simulink model "LQI_Controller"  (R2025a)
settings: Solver=FixedStepDiscrete  StartTime=0.0  StopTime=2000  FixedStep=0.01  RelTol=1e-3
values from neighbouring files (symbols this model uses):
  Ke_d = [-0.0924393948471  -0.00817730128246; 0.00819789025598  -0.0924279791075]    [LQI_params.mat]    (also in main_control.m = K_aug_d(:, 5:6))
  Kx_d = [0.12575397263  0.814001770908  0.0258937320835  0.0687846498717; -0.0126880421789  -0.0790152821896  0.235851467161  0.775518858724]    [LQI_params.mat]    (also in main_control.m = K_aug_d(:, 1:4))
  u_bar = [6.60003195923 9.28189672086]    [LQI_params.mat]    (also in linearize_4tanks.m = reshape(z_opt(5:6), [2, 1]))
  x_bar = [24.6597369405 10 3.03378366821 10]    [LQI_params.mat]    (also in linearize_4tanks.m = reshape(z_opt(1:4), [4, 1]))
  xv = 0:0.05:18    [main_control.m]
  ygamma1 = gamma1_fcn(xv)    [main_control.m]
  ygamma2 = gamma2_fcn(xv)    [main_control.m]
  yk1 = k1_fcn(xv)    [main_control.m]
  yk2 = k2_fcn(xv)    [main_control.m]
undefined symbols (not defined in the file or in its folder): AA, DiscIntNeverNeededParam
libraries: simulink x2, simulink_extras x2
settings Model: Creator=oguzhanenes  LastModifiedBy=oguzhanenes

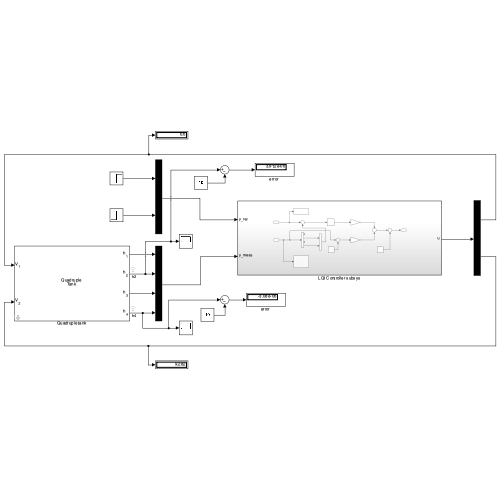
[thumbnail: Simulink's stored preview of the top-level diagram]
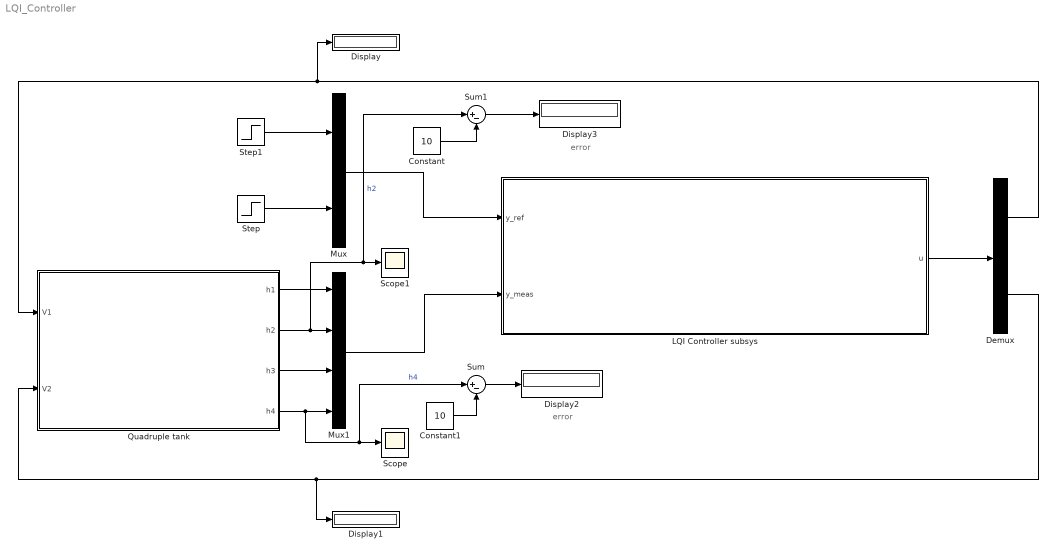
== system LQI_Controller ==
  note: error
  note: error
  Constant : Constant  Value=10
  Constant1 : Constant  Value=10
  Demux : Demux  Outputs=2
  Display{,1..3} (4 alike) : Display
  LQI Controller subsys : Subsystem
  Mux : Mux  Inputs=2
  Mux1 : Mux
  Quadruple tank : Subsystem  mask{h_0=x_bar, A=AA, S=(4.44 / 2)^2 * pi * ones(1, 4), g=981}
      mask prompts: h_0 "Initial level"; A "Outlet section"; S "Tank section"; g "Gravity"
      mask DialogControl h_0 Tooltip: [cm]
      mask DialogControl A Tooltip: [cm^2]
      mask DialogControl S Tooltip: [cm^2]
      mask DialogControl g Tooltip: [cm/s^2]
      mask Display:
      | disp('Quadruple\nTank');
      | port_label('input', 1, 'V_1', 'interpreter', 'tex');
      | port_label('input', 2, 'V_2', 'interpreter', 'tex');
      | port_label('output', 1, 'h_1', 'interpreter', 'tex');
      | port_label('output', 2, 'h_2', 'interpreter', 'tex');
      | port_label('output', 3, 'h_3', 'interpreter', 'tex');
      | port_label('output', 4, 'h_4', 'interpreter', 'tex');
  Scope : Scope
      settings: ActiveDisplayYMinimum=-838.37574082591277  ActiveDisplayYMaximum=411.67749053415992
  Scope1 : Scope
      settings: ActiveDisplayYMinimum=9.94619790425928  ActiveDisplayYMaximum=10.03798510174054
  Step : Step  Time=500  Before=10  After=10  SampleTime=0
  Step1 : Step  Time=500  Before=10  After=10  SampleTime=0
  Sum : Sum  Inputs=|+-
  Sum1 : Sum  Inputs=|+-
  wires:
  Step/1 -> Mux/2
  Mux1/1 -> LQI Controller subsys/2(y_meas)
  Mux/1 -> LQI Controller subsys/1(y_ref)
  Step1/1 -> Mux/1
  LQI Controller subsys/1(u) -> Demux/1
  Quadruple tank/1(h1) -> Mux1/1
  Quadruple tank/2(h2) -> Sum1/1, Scope1/1, Mux1/2  "h2"
  Quadruple tank/3(h3) -> Mux1/3
  Quadruple tank/4(h4) -> Sum/1, Scope/1, Mux1/4  "h4"
  Demux/1 -> Display/1, Quadruple tank/1(V1)
  Demux/2 -> Quadruple tank/2(V2), Display1/1
  Sum1/1 -> Display3/1
  Constant/1 -> Sum1/2
  Constant1/1 -> Sum/2
  Sum/1 -> Display2/1

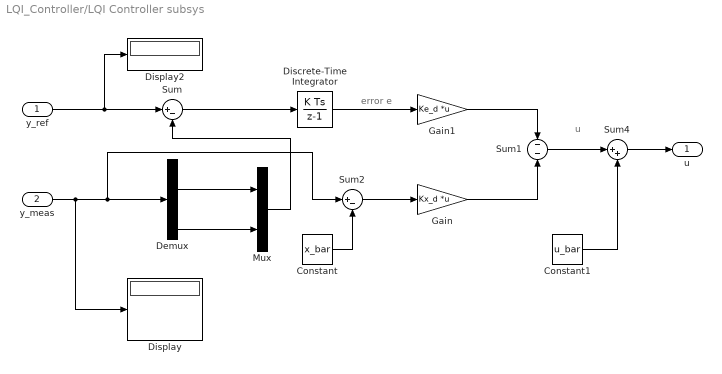
== system LQI_Controller/LQI Controller subsys ==
  note: u
  note: error e
  y_ref : Inport
  y_meas : Inport  Port=2
  Constant : Constant  Value=x_bar
  Constant1 : Constant  Value=u_bar
  Demux : Demux
  Discrete-Time Integrator : DiscreteIntegrator  SampleTime=0.01  ICPrevOutput=DiscIntNeverNeededParam  ICPrevScaledInput=DiscIntNeverNeededParam
  Display : Display
  Display2 : Display
  Gain : Gain  Gain=Kx_d  Multiplication=Matrix(K*u) (u vector)
  Gain1 : Gain  Gain=Ke_d  Multiplication=Matrix(K*u) (u vector)
  Mux : Mux  Inputs=2
  Sum : Sum  Inputs=|+-
  Sum1 : Sum  Inputs=--
  Sum2 : Sum  Inputs=|+-
  Sum4 : Sum  Inputs=|++
  u : Outport
  wires:
  y_ref/1 -> Display2/1, Sum/1
  Discrete-Time Integrator/1 -> Gain1/1
  Gain/1 -> Sum1/2
  Constant1/1 -> Sum4/2
  Sum1/1 -> Sum4/1
  Sum4/1 -> u/1
  y_meas/1 -> Display/1, Sum2/1, Demux/1
  Demux/2 -> Mux/1
  Demux/4 -> Mux/2
  Mux/1 -> Sum/2
  Sum2/1 -> Gain/1
  Constant/1 -> Sum2/2
  Gain1/1 -> Sum1/1
  Sum/1 -> Discrete-Time Integrator/1

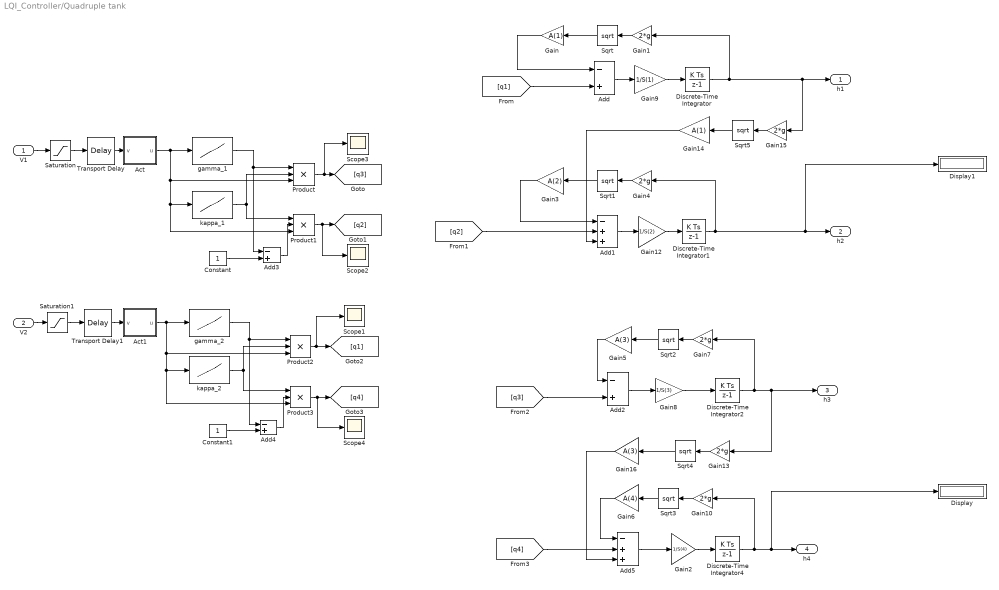
== system LQI_Controller/Quadruple tank ==
  V1 : Inport
  V2 : Inport  Port=2
  Act : Subsystem
  Act1 : Subsystem
  Add{,2..4} (4 alike) : Sum  Inputs=-+
  Add1 : Sum  Inputs=-++
  Add5 : Sum  Inputs=-++
  Constant : Constant
  Constant1 : Constant
  Discrete-Time Integrator{,1..2,4} (4 alike) : DiscreteIntegrator  SampleTime=0.01  ICPrevOutput=DiscIntNeverNeededParam  ICPrevScaledInput=DiscIntNeverNeededParam
  Display : Display
  Display1 : Display
  Gain : Gain  Gain=A(1)
  Gain{1,4,7,10,13,15} (6 alike) : Gain  Gain=2*g
  Gain12 : Gain  Gain=1/S(2)
  Gain14 : Gain  Gain=A(1)
  Gain16 : Gain  Gain=A(3)
  Gain2 : Gain  Gain=1/S(4)
  Gain3 : Gain  Gain=A(2)
  Gain5 : Gain  Gain=A(3)
  Gain6 : Gain  Gain=A(4)
  Gain8 : Gain  Gain=1/S(3)
  Gain9 : Gain  Gain=1/S(1)
  Product{,1..3} (4 alike) : Product  Inputs=3
  Saturation : Saturate  UpperLimit=18  LowerLimit=0
  Saturation1 : Saturate  UpperLimit=18  LowerLimit=0
  Scope{1..4} (4 alike) : Scope
      Scope1 settings: ActiveDisplayYMinimum=11.376007158286937  ActiveDisplayYMaximum=13.577873212532571  DataLoggingVariableName=ScopeData8
      Scope2 settings: ActiveDisplayYMinimum=11.818564666910888  ActiveDisplayYMaximum=17.795761187368054  DataLoggingVariableName=ScopeData6
      Scope3 settings: ActiveDisplayYMinimum=4.2044390084114323  ActiveDisplayYMaximum=5.0782234156834081  DataLoggingVariableName=ScopeData7
      Scope4 settings: ActiveDisplayYMinimum=16.03502727377742  ActiveDisplayYMaximum=37.82270118718629  DataLoggingVariableName=ScopeData9
  Sqrt{,1..5} (6 alike) : Sqrt
  Transport Delay : TransportDelay  DelayTime=2
  Transport Delay1 : TransportDelay  DelayTime=2
  gamma_1 : Lookup_n-D  NumberOfTableDimensions=1  BreakpointsForDimension1=xv  Table=ygamma1  ExtrapMethod=Clip  UseLastTableValue=on  InternalRulePriority=Speed  RndMeth=Simplest
  gamma_2 : Lookup_n-D  NumberOfTableDimensions=1  BreakpointsForDimension1=xv  Table=ygamma2  ExtrapMethod=Clip  UseLastTableValue=on  InternalRulePriority=Speed  RndMeth=Simplest
  kappa_1 : Lookup_n-D  NumberOfTableDimensions=1  BreakpointsForDimension1=xv  Table=yk1  ExtrapMethod=Clip  UseLastTableValue=on  InternalRulePriority=Speed  RndMeth=Simplest
  kappa_2 : Lookup_n-D  NumberOfTableDimensions=1  BreakpointsForDimension1=xv  Table=yk2  ExtrapMethod=Clip  UseLastTableValue=on  InternalRulePriority=Speed  RndMeth=Simplest
  h1 : Outport
  h2 : Outport  Port=2
  h3 : Outport  Port=3
  h4 : Outport  Port=4
  wires:
  Discrete-Time Integrator/1 -> Gain15/1, h1/1, Gain1/1
  Gain1/1 -> Sqrt/1
  Sqrt/1 -> Gain/1
  Gain/1 -> Add/1
  [q1] -> Add/2
  Add1/1 -> Gain12/1
  Gain4/1 -> Sqrt1/1
  Add2/1 -> Gain8/1
  Gain7/1 -> Sqrt2/1
  Sqrt2/1 -> Gain5/1
  Gain6/1 -> Add5/1
  Sqrt3/1 -> Gain6/1
  Gain10/1 -> Sqrt3/1
  Discrete-Time Integrator4/1 -> Display/1, h4/1, Gain10/1
  [q4] -> Add5/2
  Sqrt4/1 -> Gain16/1
  Gain13/1 -> Sqrt4/1
  Discrete-Time Integrator2/1 -> h3/1, Gain13/1, Gain7/1
  Sqrt1/1 -> Gain3/1
  Gain3/1 -> Add1/1
  Gain5/1 -> Add2/1
  Gain15/1 -> Sqrt5/1
  Sqrt5/1 -> Gain14/1
  Gain14/1 -> Add1/3
  [q2] -> Add1/2
  [q3] -> Add2/2
  Gain16/1 -> Add5/3
  gamma_1/1 -> Add3/1, Product/1
  Constant/1 -> Add3/2
  kappa_1/1 -> Product/2, Product1/1
  Add3/1 -> Product1/2
  Product/1 -> Scope3/1, [q3]
  Product1/1 -> Scope2/1, [q2]
  kappa_2/1 -> Product3/1, Product2/2
  Product2/1 -> Scope1/1, [q1]
  Constant1/1 -> Add4/2
  gamma_2/1 -> Add4/1, Product2/1
  Product3/1 -> Scope4/1, [q4]
  Add4/1 -> Product3/2
  Gain12/1 -> Discrete-Time Integrator1/1
  Add/1 -> Gain9/1
  Gain9/1 -> Discrete-Time Integrator/1
  Gain8/1 -> Discrete-Time Integrator2/1
  Add5/1 -> Gain2/1
  Gain2/1 -> Discrete-Time Integrator4/1
  Act/1(u) -> gamma_1/1, Product/3, kappa_1/1, Product1/3
  Act1/1(u) -> gamma_2/1, Product2/3, kappa_2/1, Product3/3
  Transport Delay/1 -> Act/1(v)
  V1/1 -> Saturation/1
  Saturation/1 -> Transport Delay/1
  Saturation1/1 -> Transport Delay1/1
  V2/1 -> Saturation1/1
  Transport Delay1/1 -> Act1/1(v)
  Discrete-Time Integrator1/1 -> Gain4/1, Display1/1, h2/1

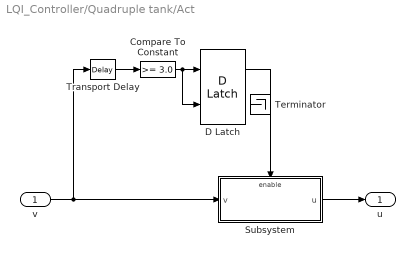
== system LQI_Controller/Quadruple tank/Act ==
  v : Inport
  Compare To Constant : simulink/Logic and Bit Operations/Compare To Constant  relop=>=  const=3.0  OutDataTypeStr=boolean
  D Latch : simulink_extras/Flip Flops/D Latch
  Subsystem : Subsystem
  Terminator : Terminator
  Transport Delay : TransportDelay  DelayTime=4
  u : Outport
  wires:
  v/1 -> Transport Delay/1, Subsystem/1(v)
  D Latch/1 -> Subsystem/Enable
  Subsystem/1(u) -> u/1
  Transport Delay/1 -> Compare To Constant/1
  Compare To Constant/1 -> D Latch/2, D Latch/1

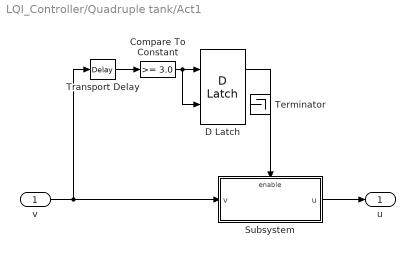
== system LQI_Controller/Quadruple tank/Act1 ==
  v : Inport
  Compare To Constant : simulink/Logic and Bit Operations/Compare To Constant  relop=>=  const=3.0  OutDataTypeStr=boolean
  D Latch : simulink_extras/Flip Flops/D Latch
  Subsystem : Subsystem
  Terminator : Terminator
  Transport Delay : TransportDelay  DelayTime=4
  u : Outport
  wires:
  v/1 -> Transport Delay/1, Subsystem/1(v)
  D Latch/1 -> Subsystem/Enable
  Subsystem/1(u) -> u/1
  Transport Delay/1 -> Compare To Constant/1
  Compare To Constant/1 -> D Latch/2, D Latch/1

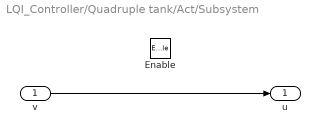
== system LQI_Controller/Quadruple tank/Act/Subsystem ==
  v : Inport
  Enable : EnablePort
  u : Outport
  wires:
  v/1 -> u/1

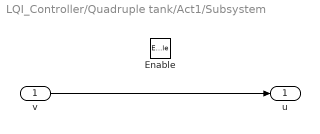
== system LQI_Controller/Quadruple tank/Act1/Subsystem ==
  v : Inport
  Enable : EnablePort
  u : Outport
  wires:
  v/1 -> u/1
